simulink library "ZH_Z"  (R2025a)
settings: Solver=VariableStepAuto  StartTime=0.0  StopTime=10.0  RelTol=1e-3
values from neighbouring files (symbols this model uses):
  C = tau^2/L    (= 1.25e-06)    [C_ZH_Z5.m]
undefined symbols (not defined in the file or in its folder): B
libraries: simulink_extras x1, M_MK x1
settings Model: Creator=Szalay  LastModifiedBy=Szalay

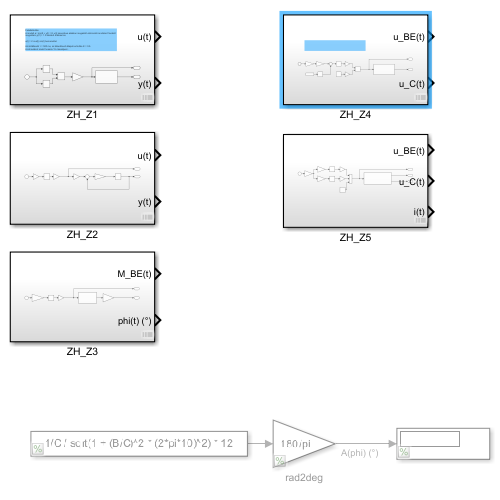
[thumbnail: Simulink's stored preview of the top-level diagram]
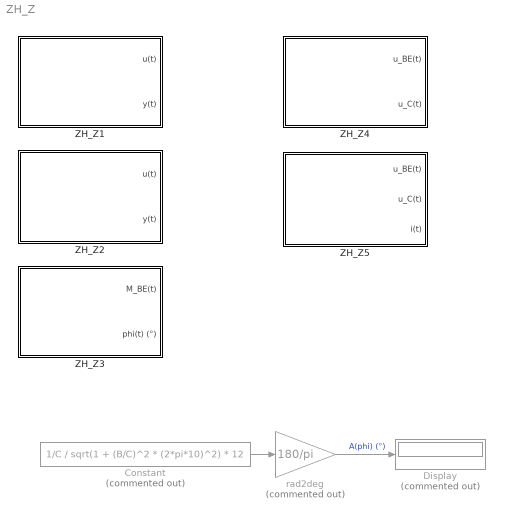
== system ZH_Z ==
  Constant : Constant  Commented=on  Value=1/C / sqrt(1 + (B/C)^2 * (2*pi*10)^2) * 12
  Display : Display  Commented=on
  ZH_Z1 : Subsystem
  ZH_Z2 : Subsystem
  ZH_Z3 : Subsystem
  ZH_Z4 : Subsystem
  ZH_Z5 : Subsystem
  rad2deg : Gain  Commented=on  Gain=180/pi
  wires:
  rad2deg/1 -> Display/1  "A(phi) (°)"
  Constant/1 -> rad2deg/1

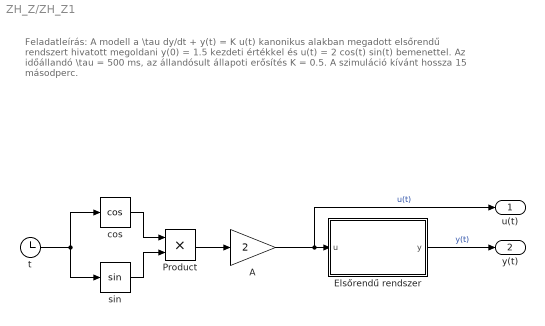
== system ZH_Z/ZH_Z1 ==
  note: Feladatleírás:
      | A modell a \tau dy/dt + y(t) = K u(t) kanonikus alakban megadott elsőrendű rendszert hivatott
      | megoldani y(0) = 1.5 kezdeti értékkel és
      |
      | u(t) = 2 cos(t) sin(t) bemenettel.
      |
      | Az időállandó \tau = 500 ms, az állandósult állapoti erősítés K = 0.5.
      | A szimuláció kívánt hossza 15 másodperc.
  A : Gain  Gain=2
  Elsőrendű rendszer : Subsystem  mask(Elsőrendű rendszer){K=0.5, tau=500e-3, y_0=1.5}
      mask prompts: K "Állandósult állapoti erősítés"; tau "Időállandó (s)"; y_0 "A kimenet kezdeti értéke"
      mask help: A lineáris közönséges elsőfokú differenciálegyenlettel jellemzett rendszer modellje.
      mask DialogControl ParameterGroupVar Prompt: Rendszerparaméterek
      mask DialogControl Container3 Prompt: Kezdeti érték
  Product : Product
  cos : Trigonometry  Operator=cos
  sin : Trigonometry
  t : Clock
  u(t) : Outport
  y(t) : Outport  Port=2
  wires:
  Elsőrendű rendszer/1(y) -> y(t)/1  "y(t)"
  A/1 -> u(t)/1, Elsőrendű rendszer/1(u)  "u(t)"
  t/1 -> cos/1, sin/1
  Product/1 -> A/1
  cos/1 -> Product/1
  sin/1 -> Product/2

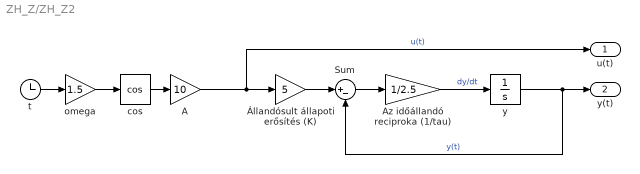
== system ZH_Z/ZH_Z2 ==
  A : Gain  Gain=10
  Az időállandó reciproka (1/tau) : Gain  Gain=1/2.5
  Sum : Sum  Inputs=|+-
  cos : Trigonometry  Operator=cos
  omega : Gain  Gain=1.5
  t : Clock
  y : Integrator  InitialCondition=-20
  Állandósult állapoti erősítés (K) : Gain  Gain=5
  u(t) : Outport
  y(t) : Outport  Port=2
  wires:
  Állandósult állapoti erősítés (K)/1 -> Sum/1
  A/1 -> u(t)/1, Állandósult állapoti erősítés (K)/1  "u(t)"
  Sum/1 -> Az időállandó reciproka (1/tau)/1
  y/1 -> y(t)/1, Sum/2  "y(t)"
  cos/1 -> A/1
  t/1 -> omega/1
  Az időállandó reciproka (1/tau)/1 -> y/1  "dy/dt"
  omega/1 -> cos/1

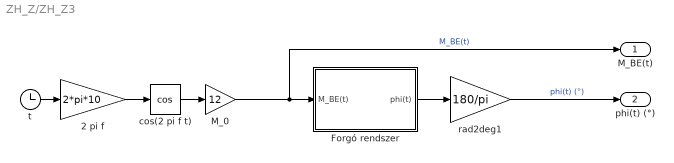
== system ZH_Z/ZH_Z3 ==
  2 pi f : Gain  Gain=2*pi*10
  Forgó rendszer : Subsystem  mask(Forgó rendszer){B=0.1, C=0.5, phi_0=45}
      mask prompts: B "Forgási súrlódási együttható"; C "Csavarási rugómerevség"; phi_0 "Kezdeti szöghelyzet (°)"
      mask DialogControl ParameterGroupVar Prompt: Rendszerparaméter
      mask DialogControl Container3 Prompt: Kezdeti érték
  M_0 : Gain  Gain=12
  cos(2 pi f t) : Trigonometry  Operator=cos
  rad2deg1 : Gain  Gain=180/pi
  t : Clock
  M_BE(t) : Outport
  phi(t) (°) : Outport  Port=2
  wires:
  cos(2 pi f t)/1 -> M_0/1
  M_0/1 -> M_BE(t)/1, Forgó rendszer/1(M_BE(t))  "M_BE(t)"
  t/1 -> 2 pi f/1
  Forgó rendszer/1(phi(t)) -> rad2deg1/1
  2 pi f/1 -> cos(2 pi f t)/1
  rad2deg1/1 -> phi(t) (°)/1  "phi(t) (°)"

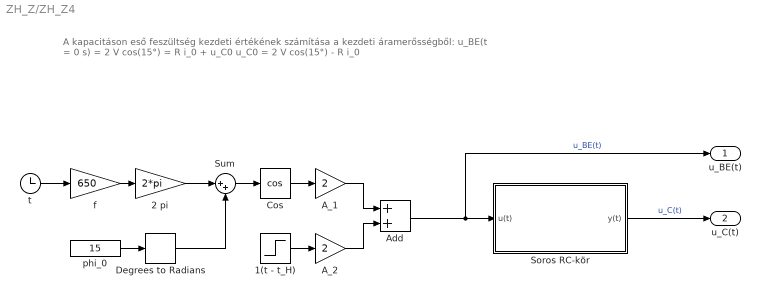
== system ZH_Z/ZH_Z4 ==
  note: A kapacitáson eső feszültség kezdeti értékének számítása a kezdeti áramerősségből:
      |
      | u_BE(t = 0 s) = 2 V cos(15°) = R i_0 + u_C0
      |
      | u_C0 = 2 V cos(15°) - R i_0
  1(t - t_H) : Step  Time=10e-3  SampleTime=0
  2 pi : Gain  Gain=2*pi
  A_1 : Gain  Gain=2
  A_2 : Gain  Gain=2
  Add : Sum
  Cos : Trigonometry  Operator=cos
  Degrees to Radians : simulink_extras/Transformations/Degrees to Radians
  Soros RC-kör : Subsystem  mask(Soros RC-kör){R=5600, C=33e-9, u_C0=2*cos(deg2rad(15)) - 5600*1e-3}
      mask prompts: R "Ellenállás (Ohm)"; C "Kapacitás (F)"; u_C0 "A kapacitás kezdeti feszültsége"
      mask help: A soros RC-kör modellje.
      mask DialogControl ParameterGroupVar Prompt: Rendszerparaméterek
      mask DialogControl Container3 Prompt: Kezdeti érték
      mask Display:
      | % Csatlakozók
      | port_label('input', 1, '{\itu}_{BE}(t)', 'texmode', 'on');
      | port_label('output', 1, '{\itu}_C(t)', 'texmode', 'on');
      | 
      | R = str2double(get_param(gcb, 'R'));
      | C = str2double(get_param(gcb, 'C'));
      | 
      | % Felirat
      | text(0.5, 0.5, ...
      |     sprintf('Soros RC-kör\n\\tau = %.3g \\mus', 1e6*R*C), ...
      |     'HorizontalAlignment', 'center', ...
      |     'Interpreter', 'tex' ...
      |     );
  Sum : Sum  Inputs=|++
  f : Gain  Gain=650
  phi_0 : Constant  Value=15
  t : Clock
  u_BE(t) : Outport
  u_C(t) : Outport  Port=2
  wires:
  t/1 -> f/1
  Degrees to Radians/1 -> Sum/2
  Cos/1 -> A_1/1
  A_2/1 -> Add/2
  Sum/1 -> Cos/1
  f/1 -> 2 pi/1
  Soros RC-kör/1(y(t)) -> u_C(t)/1  "u_C(t)"
  A_1/1 -> Add/1
  Add/1 -> Soros RC-kör/1(u(t)), u_BE(t)/1  "u_BE(t)"
  phi_0/1 -> Degrees to Radians/1
  1(t - t_H)/1 -> A_2/1
  2 pi/1 -> Sum/1

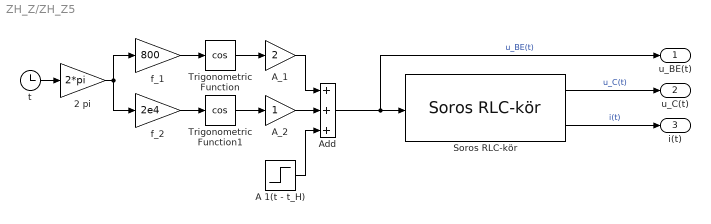
== system ZH_Z/ZH_Z5 ==
  2 pi : Gain  Gain=2*pi
  A 1(t - t_H) : Step  Time=5e-3  After=5  SampleTime=0
  A_1 : Gain  Gain=2
  A_2 : Gain
  Add : Sum  Inputs=+++
  Soros RLC-kör : M_MK/Soros RLC-kör  L=500e-6  R=2  tau=25e-6  u_C0=1  i_0=-200e-3
  Trigonometric Function : Trigonometry  Operator=cos
  Trigonometric Function1 : Trigonometry  Operator=cos
  f_1 : Gain  Gain=800
  f_2 : Gain  Gain=2e4
  t : Clock
  u_BE(t) : Outport
  u_C(t) : Outport  Port=2
  i(t) : Outport  Port=3
  wires:
  Trigonometric Function1/1 -> A_2/1
  Add/1 -> u_BE(t)/1, Soros RLC-kör/1  "u_BE(t)"
  A_2/1 -> Add/2
  A 1(t - t_H)/1 -> Add/3
  A_1/1 -> Add/1
  Soros RLC-kör/2 -> i(t)/1  "i(t)"
  2 pi/1 -> f_1/1, f_2/1
  Trigonometric Function/1 -> A_1/1
  f_2/1 -> Trigonometric Function1/1
  t/1 -> 2 pi/1
  f_1/1 -> Trigonometric Function/1
  Soros RLC-kör/1 -> u_C(t)/1  "u_C(t)"

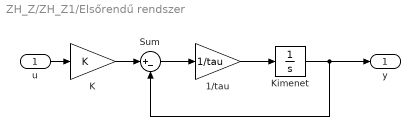
== system ZH_Z/ZH_Z1/Elsőrendű rendszer ==
  u : Inport
  1/tau : Gain  Gain=1/tau
  K : Gain  Gain=K
  Kimenet : Integrator  InitialCondition=y_0
  Sum : Sum  Inputs=|+-
  y : Outport
  wires:
  Kimenet/1 -> y/1, Sum/2
  K/1 -> Sum/1
  1/tau/1 -> Kimenet/1
  Sum/1 -> 1/tau/1
  u/1 -> K/1

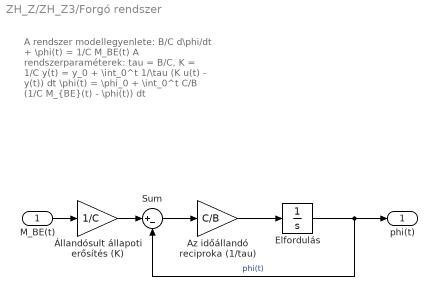
== system ZH_Z/ZH_Z3/Forgó rendszer ==
  note: A rendszer modellegyenlete:
      |
      | B/C d\phi/dt + \phi(t) = 1/C M_BE(t)
      |
      | A rendszerparaméterek:
      | tau = B/C, K = 1/C
      |
      | y(t) = y_0 + \int_0^t 1/\tau (K u(t) - y(t)) dt
      |
      | \phi(t) = \phi_0 + \int_0^t C/B (1/C M_{BE}(t) - \phi(t)) dt
  M_BE(t) : Inport
  Az időállandó reciproka (1/tau) : Gain  Gain=C/B
  Elfordulás : Integrator  InitialCondition=phi_0/180*2*pi
  Sum : Sum  Inputs=|+-
  Állandósult állapoti erősítés (K) : Gain  Gain=1/C
  phi(t) : Outport
  wires:
  Sum/1 -> Az időállandó reciproka (1/tau)/1
  Elfordulás/1 -> phi(t)/1, Sum/2  "phi(t)"
  Az időállandó reciproka (1/tau)/1 -> Elfordulás/1
  Állandósult állapoti erősítés (K)/1 -> Sum/1
  M_BE(t)/1 -> Állandósult állapoti erősítés (K)/1

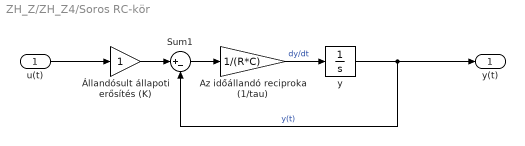
== system ZH_Z/ZH_Z4/Soros RC-kör ==
  u(t) : Inport
  Az időállandó reciproka (1/tau) : Gain  Gain=1/(R*C)
  Sum1 : Sum  Inputs=|+-
  y : Integrator  InitialCondition=u_C0
  Állandósult állapoti erősítés (K) : Gain
  y(t) : Outport
  wires:
  Az időállandó reciproka (1/tau)/1 -> y/1  "dy/dt"
  Sum1/1 -> Az időállandó reciproka (1/tau)/1
  y/1 -> y(t)/1, Sum1/2  "y(t)"
  Állandósult állapoti erősítés (K)/1 -> Sum1/1
  u(t)/1 -> Állandósult állapoti erősítés (K)/1
